simulink model "cl2"  (R2021b)
settings: Solver=FixedStepAuto  StartTime=0.0  StopTime=tf  FixedStep=ts  RelTol=1e-3
values from neighbouring files (symbols this model uses):
  a_hat_phi_ic = init + (last+init)*rand(N,1)    [problem1_test2.m]
  a_hat_x_ic = init + (last+init)*rand(N,1)    [problem1_test2.m]
  a_phi = init + (last+init)*rand(N,1)    [problem1_test2.m]
  a_x = init + (last+init)*rand(N,1)    [problem1_test2.m]
  alpha_phi = 15    [problem1_test2.m]
  alpha_x = 15    [problem1_test2.m]
  beta_phi = 15    [problem1_test2.m]
  beta_x = 15    [problem1_test2.m]
  c_phi = init + (last+init)*rand(N,1)    [problem1_test2.m]
  c_x = init + (last+init)*rand(N,1)    [problem1_test2.m]
  g = 9.8    [problem1_test2.m]
  gamma_aphi = 0.01    [problem1_test2.m]
  gamma_ax = 0.01    [problem1_test2.m]
  gamma_phi = diag(gamma_phi)    [problem1_test2.m]
  gamma_x = diag(gamma_x)    [problem1_test2.m]
  K_axp = 0.1    [problem1_test2.m]
  K_clp = 0.001*gamma_phi    [problem1_test2.m]
  K_clx = 0.001*gamma_x    [problem1_test2.m]
  l_phi = init + (last+init)*rand(N,1)    [problem1_test2.m]
  l_x = 1 + (1)*rand(N,1)    [problem1_test2.m]
  m_phi = init + (last+init)*rand(N,1)    [problem1_test2.m]
  m_x = init + (last+init)*rand(N,1)    [problem1_test2.m]
  phi_dot_ic = 0    [problem1_test2.m]
  phi_ic = init + (last+init)*rand(N,1)    [problem1_test2.m]
  s_phi = 10    [problem1_test2.m]
  s_x = 10    [problem1_test2.m]
  theta_hat_phi_ic = [init + (last+init)*rand(N,1), init + (last+init)*rand(N,1), init + (last+init)*rand(N,1)]'    [problem1_test2.m]
  theta_hat_x_ic = [init + (last+init)*rand(N,1), init + (last+init)*rand(N,1), init + (last+init)*rand(N,1), init + (last+init)*rand(N,1)]'    [problem1_test2.m]
  theta_phi = [m_phi*l_phi, m_phi*l_phi^2, c_phi]'    [problem1_test2.m]
  theta_x = [m_x, m_phi, c_x, m_phi*l_x]'    [problem1_test2.m]
  u_phi_ic = 0    [problem1_test2.m]
  u_x_ic = 0    [problem1_test2.m]
  x_dot_ic = 0    [problem1_test2.m]
  x_dotdot_ic = init + (last+init)*randn(N,1)    [problem1_test2.m]
  x_ic = init + (last+init)*randn(N,1)    [problem1_test2.m]
settings Model: Creator=kaush  LastModifiedBy=kaush
settings SolverCC: ZeroCrossAlgorithm=Adaptive

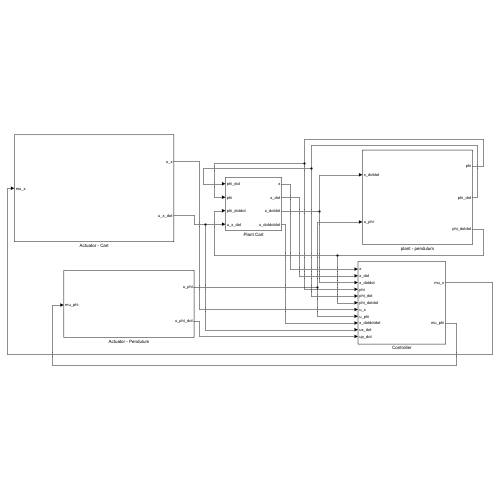
[thumbnail: Simulink's stored preview of the top-level diagram]
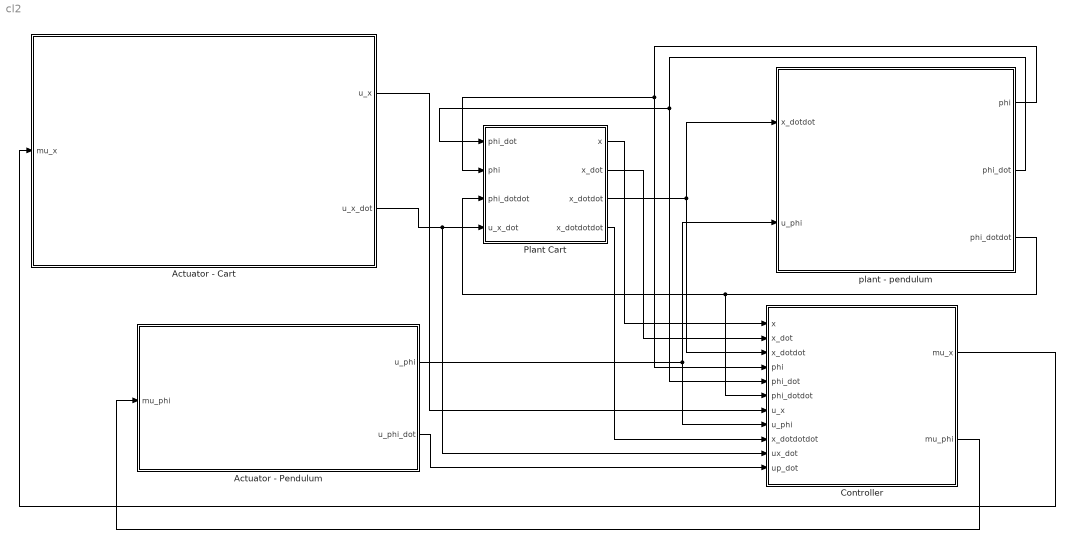
== system cl2 ==
  Actuator - Cart : Subsystem
  Actuator - Pendulum : Subsystem
  Controller : Subsystem
  Plant Cart : Subsystem
  plant - pendulum : Subsystem
  wires:
  Plant Cart/4(x_dotdotdot) -> Controller/9(x_dotdotdot)
  Controller/2(mu_phi) -> Actuator - Pendulum/1(mu_phi)
  Plant Cart/1(x) -> Controller/1(x)
  Plant Cart/3(x_dotdot) -> Controller/3(x_dotdot), plant - pendulum/1(x_dotdot)
  Actuator - Cart/2(u_x_dot) -> Controller/10(ux_dot), Plant Cart/4(u_x_dot)
  Actuator - Cart/1(u_x) -> Controller/7(u_x)
  plant - pendulum/3(phi_dotdot) -> Controller/6(phi_dotdot), Plant Cart/3(phi_dotdot)
  Actuator - Pendulum/1(u_phi) -> Controller/8(u_phi), plant - pendulum/2(u_phi)
  Plant Cart/2(x_dot) -> Controller/2(x_dot)
  plant - pendulum/2(phi_dot) -> Controller/5(phi_dot), Plant Cart/1(phi_dot)
  Controller/1(mu_x) -> Actuator - Cart/1(mu_x)
  plant - pendulum/1(phi) -> Controller/4(phi), Plant Cart/2(phi)
  Actuator - Pendulum/2(u_phi_dot) -> Controller/11(up_dot)

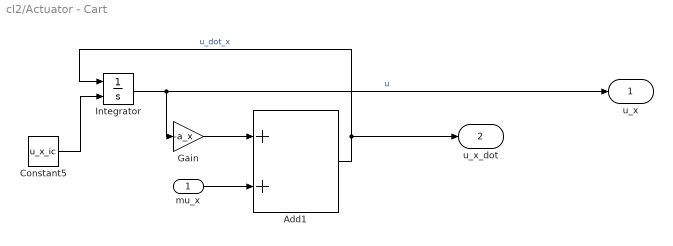
== system cl2/Actuator - Cart ==
  mu_x : Inport
  Add1 : Sum
  Constant5 : Constant  Value=u_x_ic
  Gain : Gain  Gain=-a_x
  Integrator : Integrator  InitialConditionSource=external
  u_x : Outport
  u_x_dot : Outport  Port=2
  wires:
  Add1/1 -> u_x_dot/1, Integrator/1  "u_dot_x"
  Integrator/1 -> u_x/1, Gain/1  "u"
  Gain/1 -> Add1/1
  mu_x/1 -> Add1/2
  Constant5/1 -> Integrator/2

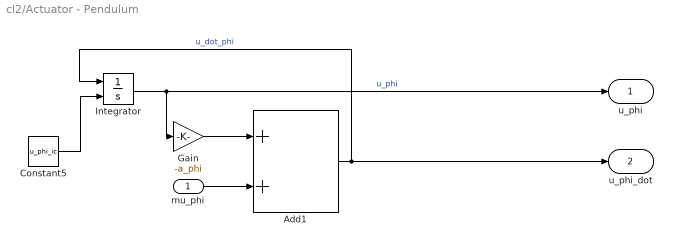
== system cl2/Actuator - Pendulum ==
  mu_phi : Inport
  Add1 : Sum
  Constant5 : Constant  Value=u_phi_ic
  Gain : Gain  Gain=-a_phi
  Integrator : Integrator  InitialConditionSource=external
  u_phi : Outport
  u_phi_dot : Outport  Port=2
  wires:
  Constant5/1 -> Integrator/2
  mu_phi/1 -> Add1/2
  Gain/1 -> Add1/1
  Integrator/1 -> Gain/1, u_phi/1  "u_phi"
  Add1/1 -> u_phi_dot/1, Integrator/1  "u_dot_phi"

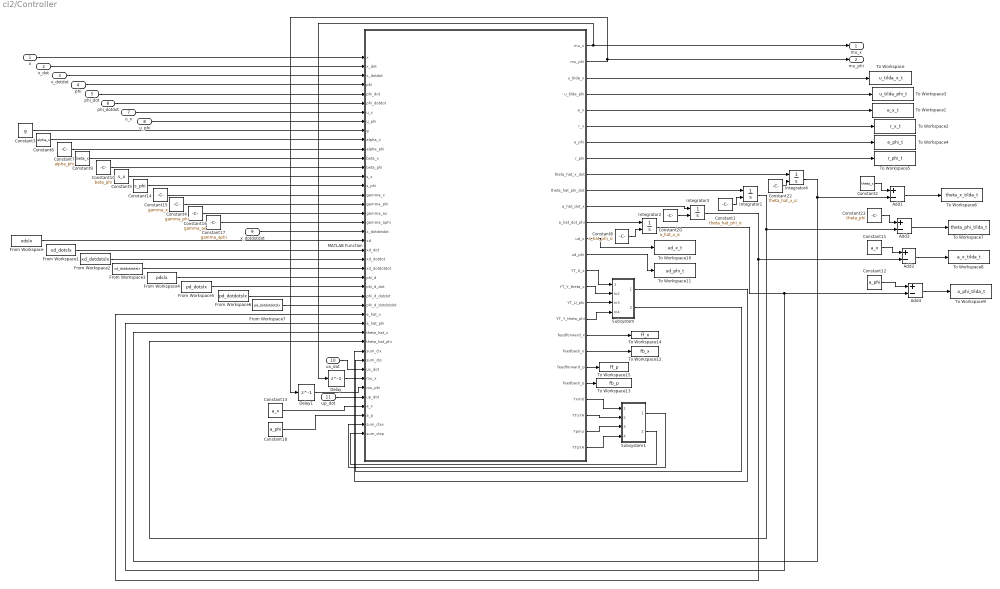
== system cl2/Controller ==
  x : Inport
  x_dot : Inport  Port=2
  x_dotdot : Inport  Port=3
  phi : Inport  Port=4
  phi_dot : Inport  Port=5
  phi_dotdot : Inport  Port=6
  u_x : Inport  Port=7
  u_phi : Inport  Port=8
  x_dotdotdot : Inport  Port=9
  ux_dot : Inport  Port=10
  up_dot : Inport  Port=11
  Add{1..4} (4 alike) : Sum  Inputs=+-
  Constant1 : Constant  Value=theta_hat_phi_ic
  Constant10 : Constant  Value=beta_phi
  Constant11 : Constant  Value=a_x
  Constant12 : Constant  Value=a_phi
  Constant13 : Constant  Value=a_x
  Constant14 : Constant  Value=s_phi
  Constant15 : Constant  Value=gamma_x
  Constant16 : Constant  Value=gamma_ax
  Constant17 : Constant  Value=gamma_aphi
  Constant18 : Constant  Value=a_phi
  Constant2 : Constant  Value=theta_x
  Constant20 : Constant  Value=a_hat_x_ic
  Constant22 : Constant  Value=theta_hat_x_ic
  Constant23 : Constant  Value=theta_phi
  Constant3 : Constant  Value=g
  Constant4 : Constant  Value=gamma_phi
  Constant5 : Constant  Value=s_x
  Constant6 : Constant  Value=alpha_x
  Constant7 : Constant  Value=alpha_phi
  Constant8 : Constant  Value=a_hat_phi_ic
  Constant9 : Constant  Value=beta_x
  Delay : Delay  DelayLength=1
  Delay1 : Delay  DelayLength=1
  From Workspace : FromWorkspace  VariableName=xdslx
  From Workspace1 : FromWorkspace  VariableName=xd_dotslx
  From Workspace2 : FromWorkspace  VariableName=xd_dotdotslx
  From Workspace3 : FromWorkspace  VariableName=xd_dotdotdotslx
  From Workspace4 : FromWorkspace  VariableName=pdslx
  From Workspace5 : FromWorkspace  VariableName=pd_dotslx
  From Workspace6 : FromWorkspace  VariableName=pd_dotdotslx
  From Workspace7 : FromWorkspace  VariableName=pd_dotdotdotslx
  Integrator{1..4} (4 alike) : Integrator  InitialConditionSource=external
  MATLAB Function : MATLAB Function  TreatAsAtomicUnit=on
  Subsystem : Subsystem
  Subsystem1 : Subsystem
  To Workspace : ToWorkspace  VariableName=u_tilda_x_t  SaveFormat=Timeseries  SampleTime=-1
  To Workspace1 : ToWorkspace  VariableName=e_x_t  SaveFormat=Timeseries  SampleTime=-1
  To Workspace10 : ToWorkspace  VariableName=ud_x_t  SaveFormat=Timeseries  SampleTime=-1
  To Workspace11 : ToWorkspace  VariableName=ud_phi_t  SaveFormat=Timeseries  SampleTime=-1
  To Workspace12 : ToWorkspace  VariableName=fb_x  SaveFormat=Timeseries  SampleTime=-1
  To Workspace13 : ToWorkspace  VariableName=fb_p  SaveFormat=Timeseries  SampleTime=-1
  To Workspace14 : ToWorkspace  VariableName=ff_x  SaveFormat=Timeseries  SampleTime=-1
  To Workspace15 : ToWorkspace  VariableName=ff_p  SaveFormat=Timeseries  SampleTime=-1
  To Workspace2 : ToWorkspace  VariableName=r_x_t  SaveFormat=Timeseries  SampleTime=-1
  To Workspace3 : ToWorkspace  VariableName=u_tilda_phi_t  SaveFormat=Timeseries  SampleTime=-1
  To Workspace4 : ToWorkspace  VariableName=e_phi_t  SaveFormat=Timeseries  SampleTime=-1
  To Workspace5 : ToWorkspace  VariableName=r_phi_t  SaveFormat=Timeseries  SampleTime=-1
  To Workspace6 : ToWorkspace  VariableName=theta_x_tilda_t  SaveFormat=Timeseries  SampleTime=-1
  To Workspace7 : ToWorkspace  VariableName=theta_phi_tilda_t  SaveFormat=Timeseries  SampleTime=-1
  To Workspace8 : ToWorkspace  VariableName=a_x_tilda_t  SaveFormat=Timeseries  SampleTime=-1
  To Workspace9 : ToWorkspace  VariableName=a_phi_tilda_t  SaveFormat=Timeseries  SampleTime=-1
  mu_x : Outport
  mu_phi : Outport  Port=2
  wires:
  u_x/1 -> MATLAB Function/7(u_x)
  phi/1 -> MATLAB Function/4(phi)
  x_dotdot/1 -> MATLAB Function/3(x_dotdot)
  u_phi/1 -> MATLAB Function/8(u_phi)
  x_dot/1 -> MATLAB Function/2(x_dot)
  x/1 -> MATLAB Function/1(x)
  phi_dot/1 -> MATLAB Function/5(phi_dot)
  phi_dotdot/1 -> MATLAB Function/6(phi_dotdot)
  Constant5/1 -> MATLAB Function/14(s_x)
  Constant6/1 -> MATLAB Function/10(alpha_x)
  Constant7/1 -> MATLAB Function/11(alpha_phi)
  Constant9/1 -> MATLAB Function/12(beta_x)
  Constant10/1 -> MATLAB Function/13(beta_phi)
  Constant3/1 -> MATLAB Function/9(g)
  Constant14/1 -> MATLAB Function/15(s_phi)
  Constant15/1 -> MATLAB Function/16(gamma_x)
  Constant16/1 -> MATLAB Function/18(gamma_ax)
  Constant4/1 -> MATLAB Function/17(gamma_phi)
  Constant17/1 -> MATLAB Function/19(gamma_aphi)
  x_dotdotdot/1 -> MATLAB Function/20(x_dotdotdot)
  From Workspace/1 -> MATLAB Function/21(xd)
  From Workspace1/1 -> MATLAB Function/22(xd_dot)
  From Workspace2/1 -> MATLAB Function/23(xd_dotdot)
  From Workspace3/1 -> MATLAB Function/24(xd_dotdotdot)
  From Workspace4/1 -> MATLAB Function/25(phi_d)
  From Workspace5/1 -> MATLAB Function/26(phi_d_dot)
  From Workspace6/1 -> MATLAB Function/27(phi_d_dotdot)
  From Workspace7/1 -> MATLAB Function/28(phi_d_dotdotdot)
  MATLAB Function/5(e_x) -> To Workspace1/1
  MATLAB Function/3(u_tilda_x) -> To Workspace/1
  MATLAB Function/6(r_x) -> To Workspace2/1
  MATLAB Function/4(u_tilda_phi) -> To Workspace3/1
  MATLAB Function/8(r_phi) -> To Workspace5/1
  MATLAB Function/7(e_phi) -> To Workspace4/1
  MATLAB Function/9(theta_hat_x_dot) -> Integrator4/1
  Constant22/1 -> Integrator4/2
  Constant1/1 -> Integrator1/2
  MATLAB Function/10(theta_hat_phi_dot) -> Integrator1/1
  Constant23/1 -> Add3/1
  Integrator1/1 -> MATLAB Function/32(theta_hat_phi), Add3/2
  Integrator4/1 -> MATLAB Function/31(theta_hat_x), Add1/2
  Constant2/1 -> Add1/1
  Add1/1 -> To Workspace6/1
  Add3/1 -> To Workspace7/1
  Constant20/1 -> Integrator3/2
  MATLAB Function/11(a_hat_dot_x) -> Integrator3/1
  Constant8/1 -> Integrator2/2
  MATLAB Function/12(a_hat_dot_phi) -> Integrator2/1
  Constant11/1 -> Add2/1
  Integrator3/1 -> MATLAB Function/29(a_hat_x), Add2/2
  Constant12/1 -> Add4/1
  Integrator2/1 -> MATLAB Function/30(a_hat_phi), Add4/2
  Add2/1 -> To Workspace8/1
  Add4/1 -> To Workspace9/1
  MATLAB Function/14(ud_phi) -> To Workspace11/1
  MATLAB Function/13(ud_x) -> To Workspace10/1
  MATLAB Function/1(mu_x) -> Delay/1, mu_x/1
  MATLAB Function/2(mu_phi) -> Delay1/1, mu_phi/1
  MATLAB Function/15(YT_U_x) -> Subsystem/1(YT_U_x)
  MATLAB Function/16(YT_Y_theta_x) -> Subsystem/2(In2)
  MATLAB Function/17(YT_U_phi) -> Subsystem/3(In3)
  MATLAB Function/18(YT_Y_theta_phi) -> Subsystem/4(In4)
  Subsystem/2(sum_clp) -> MATLAB Function/34(sum_clp)
  Subsystem/1(sum_clx) -> MATLAB Function/33(sum_clx)
  MATLAB Function/19(feedforward_x) -> To Workspace14/1
  MATLAB Function/20(feedback_x) -> To Workspace12/1
  MATLAB Function/21(feedforward_p) -> To Workspace15/1
  MATLAB Function/22(feedback_p) -> To Workspace13/1
  ux_dot/1 -> MATLAB Function/35(ux_dot)
  up_dot/1 -> MATLAB Function/38(up_dot)
  Constant13/1 -> MATLAB Function/39(a_x)
  Constant18/1 -> MATLAB Function/40(a_p)
  MATLAB Function/23(YxmU) -> Subsystem1/1(Yxmu)
  MATLAB Function/24(YTxYA) -> Subsystem1/2(YTxYA)
  MATLAB Function/25(Ypmu) -> Subsystem1/3(Ypmu)
  MATLAB Function/26(YTpYA) -> Subsystem1/4(YTpYA)
  Subsystem1/1(sum_clax) -> MATLAB Function/41(sum_clax)
  Subsystem1/2(sum_clap) -> MATLAB Function/42(sum_clap)
  Delay/1 -> MATLAB Function/36("mu_x ")
  Delay1/1 -> MATLAB Function/37("mu_phi ")

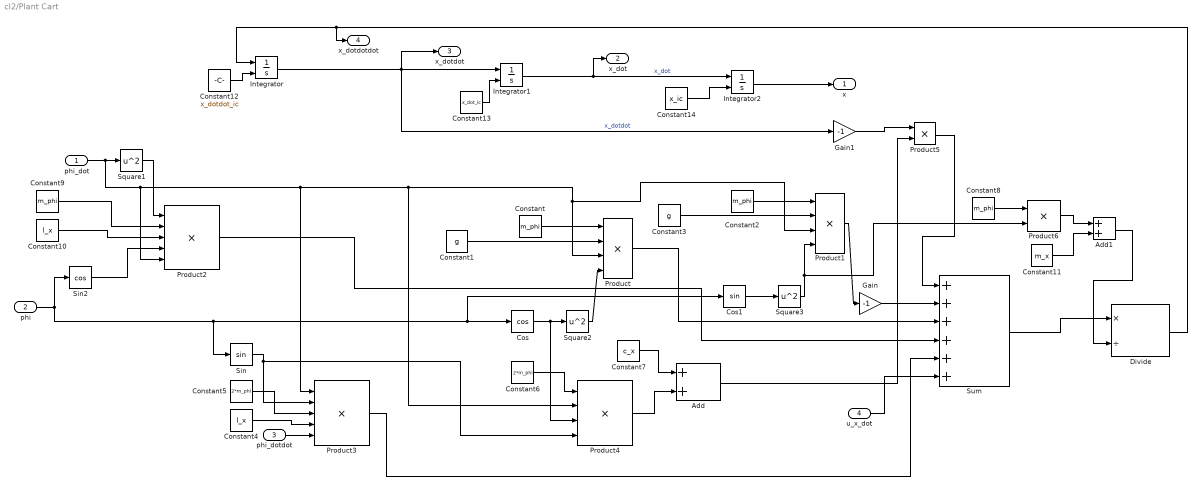
== system cl2/Plant Cart ==
  phi_dot : Inport
  phi : Inport  Port=2
  phi_dotdot : Inport  Port=3
  u_x_dot : Inport  Port=4
  Add : Sum
  Add1 : Sum
  Constant{,2,8..9} (4 alike) : Constant  Value=m_phi
  Constant1 : Constant  Value=g
  Constant10 : Constant  Value=l_x
  Constant11 : Constant  Value=m_x
  Constant12 : Constant  Value=x_dotdot_ic
  Constant13 : Constant  Value=x_dot_ic
  Constant14 : Constant  Value=x_ic
  Constant3 : Constant  Value=g
  Constant4 : Constant  Value=l_x
  Constant5 : Constant  Value=2*m_phi
  Constant6 : Constant  Value=2*m_phi
  Constant7 : Constant  Value=c_x
  Cos : Trigonometry  Operator=cos
  Cos1 : Trigonometry
  Divide : Product  Inputs=*/
  Gain : Gain  Gain=-1
  Gain1 : Gain  Gain=-1
  Integrator : Integrator  InitialConditionSource=external
  Integrator1 : Integrator  InitialConditionSource=external
  Integrator2 : Integrator  InitialConditionSource=external
  Product : Product  Inputs=4
  Product1 : Product  Inputs=4
  Product2 : Product  Inputs=5
  Product3 : Product  Inputs=5
  Product4 : Product  Inputs=4
  Product5 : Product
  Product6 : Product
  Sin : Trigonometry
  Sin2 : Trigonometry  Operator=cos
  Square1 : Math  Operator=square  SaturateOnIntegerOverflow=on
  Square2 : Math  Operator=square  SaturateOnIntegerOverflow=on
  Square3 : Math  Operator=square  SaturateOnIntegerOverflow=on
  Sum : Sum  Inputs=++++++
  x : Outport
  x_dot : Outport  Port=2
  x_dotdot : Outport  Port=3
  x_dotdotdot : Outport  Port=4
  wires:
  Divide/1 -> x_dotdotdot/1, Integrator/1
  Constant13/1 -> Integrator1/2
  Sum/1 -> Divide/1
  Add1/1 -> Divide/2
  Product6/1 -> Add1/1
  Constant12/1 -> Integrator/2
  Constant14/1 -> Integrator2/2
  Product1/1 -> Gain/1
  Constant7/1 -> Add/1
  phi_dotdot/1 -> Product3/5
  Constant6/1 -> Product4/1
  Gain/1 -> Sum/2
  Constant2/1 -> Product1/1
  Square3/1 -> Product6/2, Product1/4
  Constant11/1 -> Add1/2
  Constant3/1 -> Product1/2
  Product5/1 -> Sum/1
  Constant1/1 -> Product/2
  Square2/1 -> Product/4
  Product3/1 -> Sum/5
  Constant/1 -> Product/1
  phi/1 -> Sin/1, Cos1/1, Cos/1, Sin2/1
  u_x_dot/1 -> Sum/6
  Constant9/1 -> Product2/2
  Sin2/1 -> Product2/4
  Constant10/1 -> Product2/3
  Square1/1 -> Product2/1
  phi_dot/1 -> Product2/5, Product3/1, Product4/2, Product1/3, Product/3, Square1/1
  Integrator/1 -> Gain1/1, x_dotdot/1, Integrator1/1  "x_dotdot"
  Product2/1 -> Sum/4
  Integrator1/1 -> x_dot/1, Integrator2/1  "x_dot"
  Constant5/1 -> Product3/3
  Integrator2/1 -> x/1
  Sin/1 -> Product4/4, Product3/2
  Product/1 -> Sum/3
  Cos/1 -> Square2/1, Product4/3
  Product4/1 -> Add/2
  Add/1 -> Product5/2
  Constant8/1 -> Product6/1
  Cos1/1 -> Square3/1
  Constant4/1 -> Product3/4
  Gain1/1 -> Product5/1

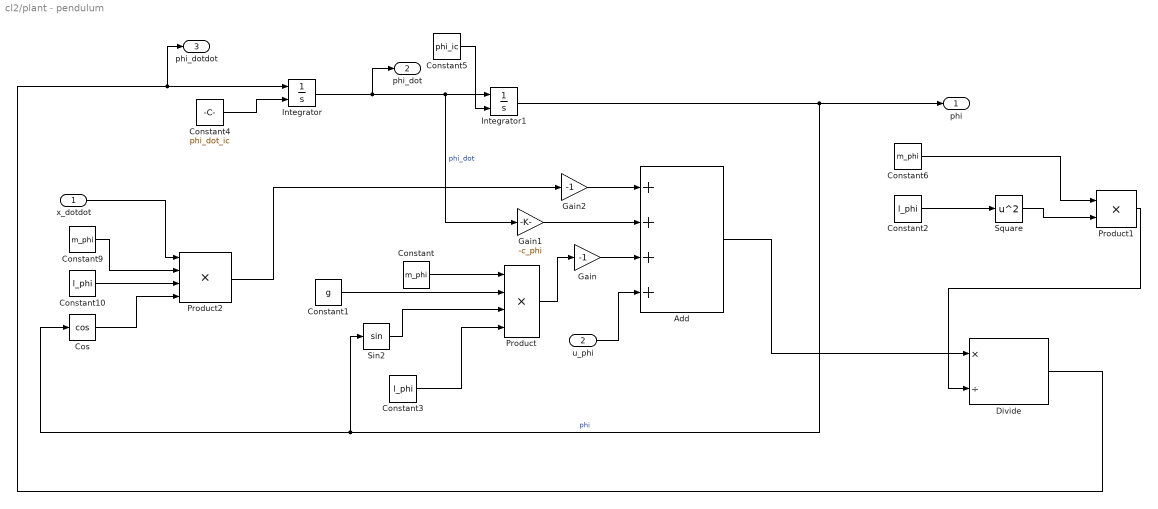
== system cl2/plant - pendulum ==
  x_dotdot : Inport
  u_phi : Inport  Port=2
  Add : Sum  Inputs=++++
  Constant : Constant  Value=m_phi
  Constant1 : Constant  Value=g
  Constant10 : Constant  Value=l_phi
  Constant2 : Constant  Value=l_phi
  Constant3 : Constant  Value=l_phi
  Constant4 : Constant  Value=phi_dot_ic
  Constant5 : Constant  Value=phi_ic
  Constant6 : Constant  Value=m_phi
  Constant9 : Constant  Value=m_phi
  Cos : Trigonometry  Operator=cos
  Divide : Product  Inputs=*/
  Gain : Gain  Gain=-1
  Gain1 : Gain  Gain=-c_phi
  Gain2 : Gain  Gain=-1
  Integrator : Integrator  InitialConditionSource=external
  Integrator1 : Integrator  InitialConditionSource=external
  Product : Product  Inputs=4
  Product1 : Product
  Product2 : Product  Inputs=4
  Sin2 : Trigonometry
  Square : Math  Operator=square  SaturateOnIntegerOverflow=on
  phi : Outport
  phi_dot : Outport  Port=2
  phi_dotdot : Outport  Port=3
  wires:
  x_dotdot/1 -> Product2/1
  Constant10/1 -> Product2/3
  Constant9/1 -> Product2/2
  Constant3/1 -> Product/4
  Gain1/1 -> Add/2
  Constant4/1 -> Integrator/2
  Product2/1 -> Gain2/1
  Sin2/1 -> Product/3
  Integrator/1 -> Gain1/1, Integrator1/1, phi_dot/1  "phi_dot"
  Constant5/1 -> Integrator1/2
  Constant1/1 -> Product/2
  Add/1 -> Divide/1
  Constant/1 -> Product/1
  u_phi/1 -> Add/4
  Integrator1/1 -> phi/1, Sin2/1, Cos/1  "phi"
  Product/1 -> Gain/1
  Gain/1 -> Add/3
  Cos/1 -> Product2/4
  Gain2/1 -> Add/1
  Constant2/1 -> Square/1
  Constant6/1 -> Product1/1
  Square/1 -> Product1/2
  Divide/1 -> Integrator/1, phi_dotdot/1
  Product1/1 -> Divide/2

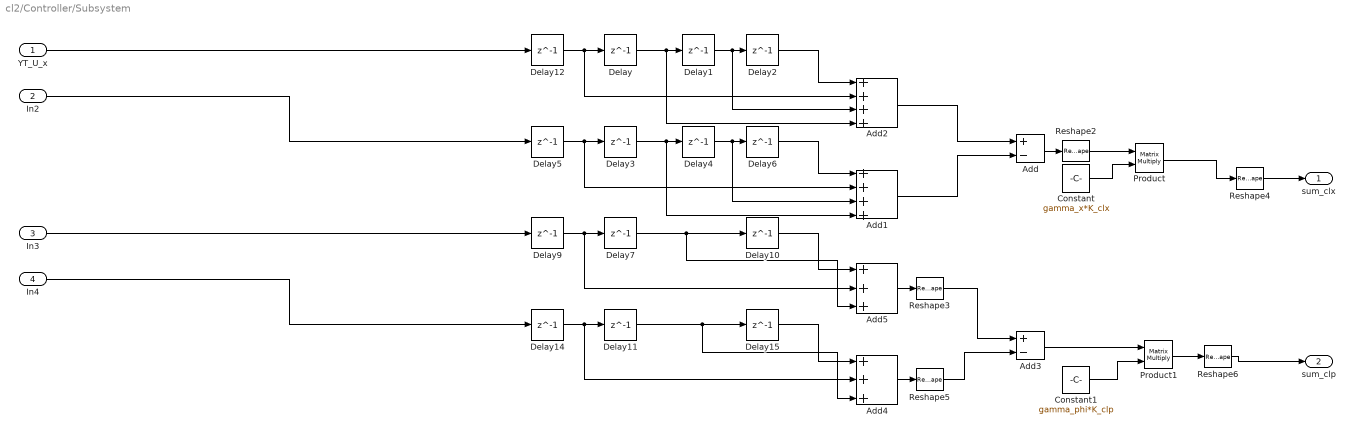
== system cl2/Controller/Subsystem ==
  YT_U_x : Inport  PortDimensions=[4,1]
  In2 : Inport  Port=2  PortDimensions=[4,1]
  In3 : Inport  Port=3  PortDimensions=[3,1]
  In4 : Inport  Port=4  PortDimensions=[3,1]
  Add : Sum  Inputs=+-
  Add1 : Sum  Inputs=++++
  Add2 : Sum  Inputs=++++
  Add3 : Sum  Inputs=+-
  Add4 : Sum  Inputs=+++
  Add5 : Sum  Inputs=+++
  Constant : Constant  Value=gamma_x*K_clx
  Constant1 : Constant  Value=gamma_phi*K_clp
  Delay{,1..2,12} (4 alike) : Delay  DelayLength=1  InitialCondition=zeros(4,1)
  Delay{3..7,9..11,14..15} (10 alike) : Delay  DelayLength=1
  Product : Product  Multiplication=Matrix(*)
  Product1 : Product  Multiplication=Matrix(*)
  Reshape2 : Reshape  OutputDimensionality=Row vector (2-D)
  Reshape3 : Reshape  OutputDimensionality=Row vector (2-D)
  Reshape4 : Reshape
  Reshape5 : Reshape  OutputDimensionality=Row vector (2-D)
  Reshape6 : Reshape
  sum_clx : Outport
  sum_clp : Outport  Port=2
  wires:
  In4/1 -> Delay14/1
  Add2/1 -> Add/1
  Delay12/1 -> Add2/2, Delay/1
  Delay/1 -> Add2/4, Delay1/1
  Product/1 -> Reshape4/1
  Delay15/1 -> Add4/1
  Add5/1 -> Reshape3/1
  Delay1/1 -> Add2/3, Delay2/1
  Delay14/1 -> Add4/2, Delay11/1
  In2/1 -> Delay5/1
  Delay10/1 -> Add5/1
  Add4/1 -> Reshape5/1
  Delay7/1 -> Delay10/1, Add5/3
  Delay9/1 -> Add5/2, Delay7/1
  Reshape3/1 -> Add3/1
  YT_U_x/1 -> Delay12/1
  Add/1 -> Reshape2/1
  In3/1 -> Delay9/1
  Add3/1 -> Product1/1
  Product1/1 -> Reshape6/1
  Delay3/1 -> Add1/4, Delay4/1
  Delay11/1 -> Delay15/1, Add4/3
  Reshape5/1 -> Add3/2
  Delay2/1 -> Add2/1
  Delay5/1 -> Add1/2, Delay3/1
  Delay4/1 -> Add1/3, Delay6/1
  Delay6/1 -> Add1/1
  Constant/1 -> Product/2
  Constant1/1 -> Product1/2
  Reshape4/1 -> sum_clx/1
  Reshape6/1 -> sum_clp/1
  Reshape2/1 -> Product/1
  Add1/1 -> Add/2

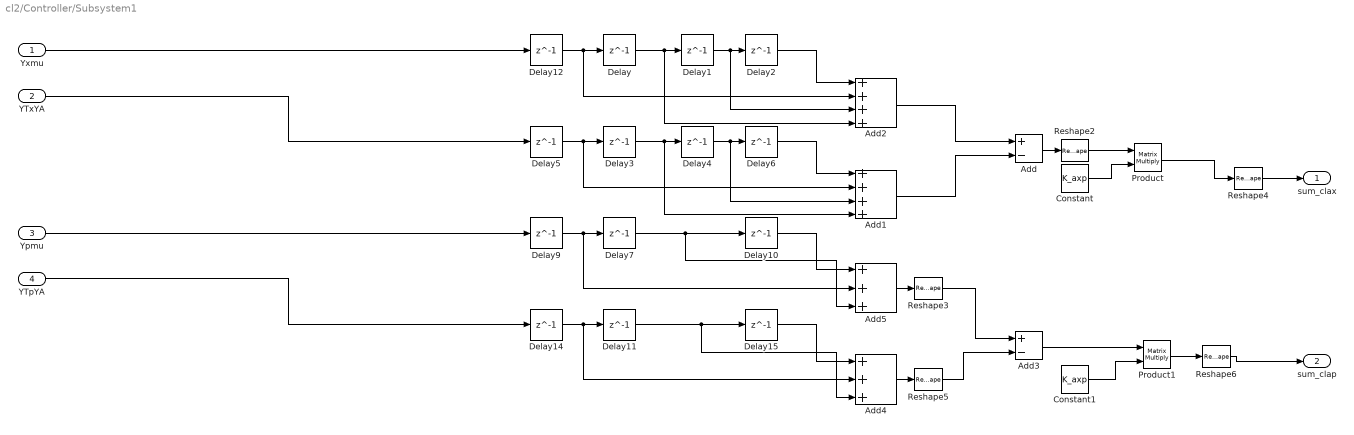
== system cl2/Controller/Subsystem1 ==
  Yxmu : Inport  PortDimensions=[1,1]
  YTxYA : Inport  Port=2  PortDimensions=[1,1]
  Ypmu : Inport  Port=3  PortDimensions=[1,1]
  YTpYA : Inport  Port=4  PortDimensions=[1,1]
  Add : Sum  Inputs=+-
  Add1 : Sum  Inputs=++++
  Add2 : Sum  Inputs=++++
  Add3 : Sum  Inputs=+-
  Add4 : Sum  Inputs=+++
  Add5 : Sum  Inputs=+++
  Constant : Constant  Value=K_axp
  Constant1 : Constant  Value=K_axp
  Delay{,1..2,12} (4 alike) : Delay  DelayLength=1  InitialCondition=zeros(1,1)
  Delay{3..7,9..11,14..15} (10 alike) : Delay  DelayLength=1
  Product : Product  Multiplication=Matrix(*)
  Product1 : Product  Multiplication=Matrix(*)
  Reshape2 : Reshape  OutputDimensionality=Row vector (2-D)
  Reshape3 : Reshape  OutputDimensionality=Row vector (2-D)
  Reshape4 : Reshape
  Reshape5 : Reshape  OutputDimensionality=Row vector (2-D)
  Reshape6 : Reshape
  sum_clax : Outport
  sum_clap : Outport  Port=2
  wires:
  YTpYA/1 -> Delay14/1
  Add2/1 -> Add/1
  Delay12/1 -> Add2/2, Delay/1
  Delay/1 -> Add2/4, Delay1/1
  Product/1 -> Reshape4/1
  Delay15/1 -> Add4/1
  Add5/1 -> Reshape3/1
  Delay1/1 -> Add2/3, Delay2/1
  Delay14/1 -> Add4/2, Delay11/1
  YTxYA/1 -> Delay5/1
  Delay10/1 -> Add5/1
  Add4/1 -> Reshape5/1
  Delay7/1 -> Delay10/1, Add5/3
  Delay9/1 -> Add5/2, Delay7/1
  Reshape3/1 -> Add3/1
  Yxmu/1 -> Delay12/1
  Add/1 -> Reshape2/1
  Ypmu/1 -> Delay9/1
  Add3/1 -> Product1/1
  Product1/1 -> Reshape6/1
  Delay3/1 -> Add1/4, Delay4/1
  Delay11/1 -> Delay15/1, Add4/3
  Reshape5/1 -> Add3/2
  Delay2/1 -> Add2/1
  Delay5/1 -> Add1/2, Delay3/1
  Delay4/1 -> Add1/3, Delay6/1
  Delay6/1 -> Add1/1
  Constant/1 -> Product/2
  Constant1/1 -> Product1/2
  Reshape4/1 -> sum_clax/1
  Reshape6/1 -> sum_clap/1
  Reshape2/1 -> Product/1
  Add1/1 -> Add/2

== matlab function cl2/Controller/MATLAB Function ==
  data: x input; mu_x output; x_dot input; mu_phi output; u_tilda_x output; u_tilda_phi output; e_x output; r_x output; e_phi output; r_phi output; theta_hat_x_dot output; theta_hat_phi_dot output; a_hat_dot_x output; a_hat_dot_phi output; ud_x output; x_dotdot input; phi input; phi_dot input; phi_dotdot input; u_x input; u_phi input; g input; alpha_x input; alpha_phi input; beta_x input; beta_phi input; s_x input; s_phi input; gamma_x input; gamma_phi input; gamma_ax input; gamma_aphi input; x_dotdotdot input; xd input; xd_dot input; xd_dotdot input; xd_dotdotdot input; phi_d input; phi_d_dot input; phi_d_dotdot input; phi_d_dotdotdot input; a_hat_x input; a_hat_phi input; theta_hat_x input; theta_hat_phi input; ud_phi output; YT_U_x output; YT_Y_theta_x output; YT_U_phi output; YT_Y_theta_phi output; sum_clx input; sum_clp input; feedforward_x output; feedback_x output; feedforward_p output; feedback_p output; ux_dot input; mu_x input; mu_phi input; up_dot input; a_x input; a_p input; YxmU output; YTxYA output; Ypmu output; YTpYA output; sum_clax input; sum_clap input
function [mu_x, mu_phi, u_tilda_x, u_tilda_phi, e_x, r_x, e_phi, r_phi, ...
    theta_hat_x_dot, theta_hat_phi_dot, a_hat_dot_x, a_hat_dot_phi, ud_x, ...
    ud_phi, YT_U_x, YT_Y_theta_x, YT_U_phi, YT_Y_theta_phi, feedforward_x, feedback_x, feedforward_p, feedback_p, YxmU, YTxYA, Ypmu, YTpYA] = fcn(x, x_dot, x_dotdot, phi, phi_dot, ...
    phi_dotdot, u_x, u_phi, g, alpha_x, alpha_phi, beta_x, beta_phi, s_x, s_phi, gamma_x, ...
    gamma_phi, gamma_ax, gamma_aphi, x_dotdotdot, xd, xd_dot, xd_dotdot, xd_dotdotdot, phi_d, ...
    phi_d_dot, phi_d_dotdot, phi_d_dotdotdot, a_hat_x, a_hat_phi, theta_hat_x, theta_hat_phi, sum_clx, sum_clp, ux_dot, mu_x, mu_phi, up_dot, a_x, a_p, sum_clax, sum_clap)
% function [mu_x, mu_phi, u_tilda_x, u_tilda_phi, e_x, r_x, e_phi, r_phi, theta_hat_x_dot, theta_hat_phi_dot, a_hat_dot_x, a_hat_dot_phi, ud_x, ud_phi, YT_U_x, YT_Y_theta_x, YT_U_phi, YT_Y_theta_phi] = fcn(x, x_dot, x_dotdot, phi, phi_dot, phi_dotdot, u_x, u_phi, g, alpha_x, alpha_phi, beta_x, beta_phi, s_x, s_phi, gamma_x, gamma_phi, gamma_ax, gamma_aphi, x_dotdotdot, xd, xd_dot, xd_dotdot, xd_dotdotdot, phi_d, phi_d_dot, phi_d_dotdot, phi_d_dotdotdot, a_hat_x, a_hat_phi, theta_hat_x, theta_hat_phi, sum_clx, sum_clp)
% function [mu_x, mu_phi, u_tilda_x, u_tilda_phi, e_x ,r_x, e_phi, r_phi, theta_hat_x_dot, theta_hat_phi_dot, a_hat_dot_x, a_hat_dot_phi, ud_x, ud_phi, YT_U_x, YT_Y_theta_x, YT_U_phi, YT_Y_theta_phi] = fcn( x, x_dot, ...
%     x_dotdot, phi, phi_dot, phi_dotdot, u_x, u_phi, g, ...
%     alpha_x, alpha_phi, beta_x, beta_phi, s_x, s_phi, gamma_x, gamma_phi, ...
%     gamma_ax, gamma_aphi, x_dotdotdot, xd, xd_dot, xd_dotdot, xd_dotdotdot, phi_d, phi_d_dot, phi_d_dotdot, phi_d_dotdotdot, a_hat_x, a_hat_phi, theta_hat_x,theta_hat_phi,sum_clx, sum_clp)
% % Cart Dynamics
% 
% sum_clx = zeros(4,1) 
% sum_clp = zeros(3,1)

mu_x = 1e-2; 
mu_phi = 1e-3; 
u_tilda_x =1e-4;
u_tilda_phi= 1e-3;
e_x =1e-3;
r_x =1e-3;
e_phi=1e-3;
r_phi=1e-3;
theta_hat_x_dot=1e-3*ones(4,1); 
theta_hat_phi_dot=1e-3*ones(3,1); 
a_hat_dot_x=1e-3; 
a_hat_dot_phi=1e-3;
ud_x=1e-3;
ud_phi=1e-3;
YT_U_x=1e-3*ones(4,1);
YT_Y_theta_x=1e-3*ones(4,1);
YT_U_phi=1e-3*ones(3,1);
YT_Y_theta_phi=1e-3*ones(3,1);



e_x = xd - x;
e_x_dot = xd_dot - x_dot;
e_x_dotdot = xd_dotdot - x_dotdot;
r_x = e_x_dot + alpha_x*e_x;
r_x_dot = e_x_dotdot + alpha_x*e_x_dot;
Y_x = [(alpha_x*e_x_dot + xd_dotdot), (sin(phi)*sin(phi)*alpha_x*e_x_dot + sin(phi)*sin(phi)*xd_dotdot + sin(phi)*cos(phi)*phi_dot*r_x - g*cos(phi)*sin(phi)), (x_dot), (-phi_dot^2*sin(phi))];
Y_x_dot = [(alpha_x*e_x_dotdot + xd_dotdotdot), (r_x*cos(phi)*cos(phi)*phi_dot^2 - r_x*sin(phi)*sin(phi)*phi_dot^2 + r_x*sin(phi)*cos(phi)*phi_dotdot + sin(phi)*cos(phi)*phi_dot*r_x_dot + alpha_x*sin(phi)*sin(phi)*e_x_dotdot + xd_dotdot*2*sin(phi)*cos(phi)*phi_dot + sin(phi)*sin(phi)*xd_dotdotdot - g*cos(phi)*cos(phi)*phi_dot + g*sin(phi)*sin(phi)*phi_dot + 2*sin(phi)*cos(phi)*phi_dot*alpha_x*e_x_dot), (x_dotdot), (-2*phi_dot*sin(phi)*phi_dotdot - phi_dot^3*cos(phi))];

Y_zx = [(x_dotdot), (sin(phi)*sin(phi)*x_dotdot - g*cos(phi)*sin(phi)), (x_dot), (-phi_dot^2*sin(phi))];
YT_U_x = Y_zx'*u_x;
YT_Y_theta_x = Y_zx'*Y_zx*theta_hat_x;


% YT_U_phi = Y_zp'*u_phi;
% YT_Y_theta_phi = Y_zp'*Y_zp*theta_hat_phi;
     
% sum_clx
K_tx = gamma_x;
theta_hat_x_dot = gamma_x*Y_x'*r_x + gamma_x*K_tx*(YT_U_x - YT_Y_theta_x) + sum_clx;
% theta_hat_x_dot =0;
feedforward_x = Y_x*theta_hat_x;
feedback_x = e_x + beta_x*r_x;
ud_x = Y_x*theta_hat_x + e_x + beta_x*r_x;
u_tilda_x = ud_x - u_x;
a_hat_dot_x = gamma_ax*u_tilda_x*u_x + sum_clax;
ud_x_dot = Y_x*theta_hat_x_dot + Y_x_dot*theta_hat_x + e_x_dot + beta_x*r_x_dot;
mu_x = ud_x_dot + a_hat_x*u_x + r_x + s_x*u_tilda_x;

%Y_cx = [ux_dot, u_x];
%theta_ax = [1, a_x]';
Y_ax = u_x;
YxmU = Y_ax'*(mu_x - ux_dot);
YTxYA = Y_ax'*Y_ax*a_hat_x;

% 
% 
% % Pendulum Dynamics 
% 
e_phi = phi_d - phi;
e_phi_dot = phi_d_dot - phi_dot;
e_phi_dotdot = phi_d_dotdot - phi_dotdot;
r_phi = e_phi_dot + alpha_phi*e_phi;
r_phi_dot = e_phi_dotdot + alpha_phi*e_phi_dot;
Y_phi = [(g*sin(phi)+cos(phi)*x_dotdot), (phi_d_dotdot + alpha_phi*e_phi_dot), phi_dot];
Y_phi_dot = [g*cos(phi)*phi_dot + x_dotdotdot*cos(phi) - x_dotdot*sin(phi)*phi_dot, alpha_phi*e_phi_dotdot + phi_d_dotdotdot, phi_dotdot];
Y_zp = [(g*sin(phi)+cos(phi)*x_dotdot), (phi_dotdot), (phi_dot)];

YT_U_phi = Y_zp'*u_phi;
YT_Y_theta_phi = Y_zp'*Y_zp*theta_hat_phi;



K_tp = gamma_phi;
theta_hat_phi_dot = gamma_phi*Y_phi'*r_phi + gamma_phi*K_tp*(YT_U_phi - YT_Y_theta_phi) + sum_clp;
%theta_hat_phi_dot = gamma_phi*Y_phi'*r_phi;
% theta_hat_phi_dot = 0;
feedforward_p = Y_phi*theta_hat_phi;
feedback_p = e_phi + beta_phi*r_phi;
ud_phi = e_phi + beta_phi*r_phi + Y_phi*theta_hat_phi;
u_tilda_phi = ud_phi - u_phi;
a_hat_dot_phi = gamma_aphi*u_tilda_phi*u_phi + sum_clap;
ud_phi_dot = Y_phi*theta_hat_phi_dot + Y_phi_dot*theta_hat_phi + e_phi_dot + beta_phi*r_phi_dot;
mu_phi = ud_phi_dot + a_hat_phi*u_phi + r_phi + s_phi*u_tilda_phi;

%Y_cp = [up_dot, u_phi];
%theta_ap = [1, a_phi]';
Y_ap = u_phi;
Ypmu = Y_ap'*mu_phi;
YTpYA = Y_ap'*Y_ap*a_hat_phi;
